simulink model "OPSID_Jawwad"  (R2023a)
settings: Solver=VariableStepAuto  StartTime=0.0  StopTime=10.0  RelTol=1e-3
values from neighbouring files (symbols this model uses):
  Kd = diag([30,30,20,20,20,20])    [parameters.m]
  Kp = diag([280,280,70,70,70,70])    [parameters.m]
libraries: robotcorelib x1
settings Model: Creator=uzair  LastModifiedBy=syedj
settings OptimizationCC: ReuseModelBlockBuffer=off

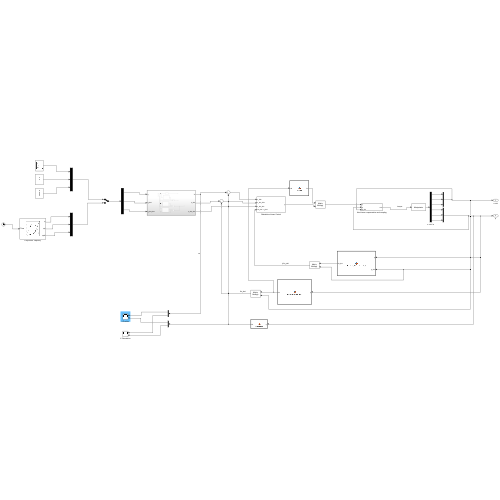
[thumbnail: Simulink's stored preview of the top-level diagram]
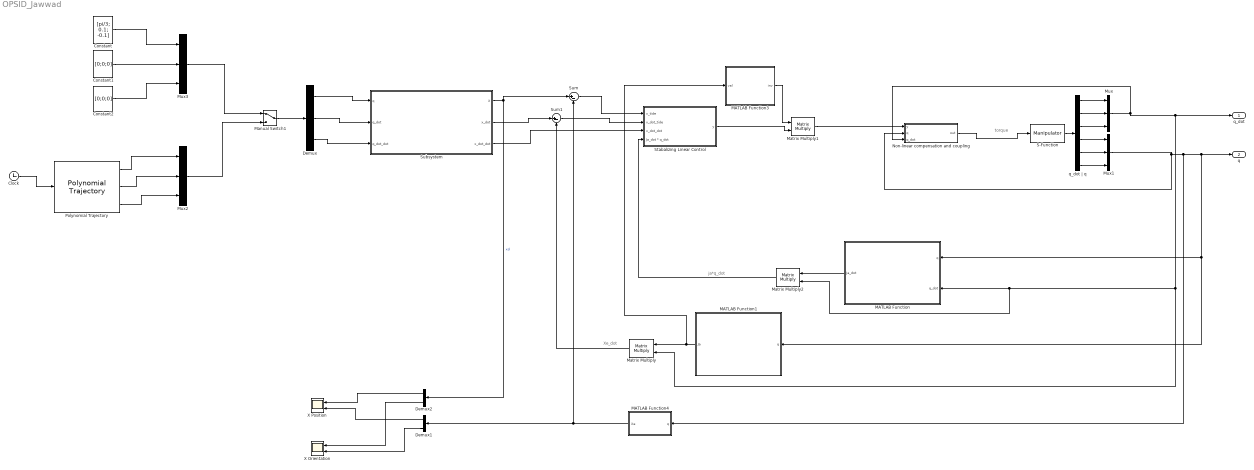
== system OPSID_Jawwad ==
  note: torque
  note: ja*q_dot
  note: Xe_dot
  Clock : Clock
  Constant : Constant  Value=[pi/3; 0.1; -0.1]  VectorParams1D=off
  Constant1 : Constant  Value=[0;0;0]  VectorParams1D=off
  Constant2 : Constant  Value=[0;0;0]  VectorParams1D=off
  Demux : Demux  Outputs=3
  Demux1 : Demux  Outputs=2
  Demux2 : Demux  Outputs=2
  MATLAB Function : MATLAB Function  TreatAsAtomicUnit=on
  MATLAB Function1 : MATLAB Function  TreatAsAtomicUnit=on
  MATLAB Function3 : MATLAB Function  TreatAsAtomicUnit=on
  MATLAB Function4 : MATLAB Function  TreatAsAtomicUnit=on
  Manual Switch1 : ManualSwitch
  Matrix Multiply : Product  Multiplication=Matrix(*)
  Matrix Multiply1 : Product  Multiplication=Matrix(*)
  Matrix Multiply2 : Product  Multiplication=Matrix(*)
  Mux{,1..3} (4 alike) : Mux  Inputs=3
  Non-linear compensation and coupling : Subsystem
  Polynomial Trajectory : robotcorelib/Polynomial Trajectory  WaypointSource=Internal  Waypoints=[pi,2*pi,3*pi; -0.2,0,-0.2; pi/2,pi,pi/2]  TimePoints=[ 0, 4, 9]  TimeInterval=[ 1, 4 ]  Method=Cubic Polynomial  ParameterSource=Internal  VelocityBoundaryCondition=zeros( 3,3 )  AccelerationBoundaryCondition=zeros( 3,3 )  SimulateUsing=Interpreted execution
  S-Function : S-Function  FunctionName=Manipulator  Parameters=params  SFunctionDeploymentMode=off  EnableBusSupport=off
  Stabalizing Linear Control : Subsystem
  Subsystem : Subsystem
  Sum : Sum  Inputs=|+-
  Sum1 : Sum  Inputs=|+-
  X Orientation : Scope  NumInputPorts=2
  X Position : Scope  NumInputPorts=2
  q_dot | q : Demux  Outputs=6
  q_dot : Outport
  q : Outport  Port=2
  wires:
  S-Function/1 -> q_dot | q/1
  q_dot | q/1 -> Mux/1
  q_dot | q/2 -> Mux/2
  q_dot | q/3 -> Mux/3
  q_dot | q/6 -> Mux1/3
  q_dot | q/5 -> Mux1/2
  q_dot | q/4 -> Mux1/1
  Mux/1 -> Matrix Multiply/2, Matrix Multiply2/2, MATLAB Function/2(q_dot), q_dot/1, Non-linear compensation and coupling/3(q_dot)
  Mux1/1 -> Non-linear compensation and coupling/2(q), MATLAB Function4/1(q), MATLAB Function1/1(q), MATLAB Function/1(q), q/1
  Sum/1 -> Stabalizing Linear Control/1(x_tide)
  Sum1/1 -> Stabalizing Linear Control/2(x_dot_tide)
  Clock/1 -> Polynomial Trajectory/1
  Non-linear compensation and coupling/1(out) -> S-Function/1
  Polynomial Trajectory/1 -> Mux2/1
  Polynomial Trajectory/2 -> Mux2/2
  Polynomial Trajectory/3 -> Mux2/3
  Constant/1 -> Mux3/1
  Constant1/1 -> Mux3/2
  Constant2/1 -> Mux3/3
  Mux3/1 -> Manual Switch1/1
  Mux2/1 -> Manual Switch1/2
  Manual Switch1/1 -> Demux/1
  Subsystem/2(x_dot) -> Sum1/1
  Subsystem/3(x_dot_dot) -> Stabalizing Linear Control/3(x_dot_dot)
  Demux/1 -> Subsystem/1(q)
  Demux/2 -> Subsystem/2(q_dot)
  Demux/3 -> Subsystem/3(q_dot_dot)
  MATLAB Function1/1(Ja) -> MATLAB Function3/1(val), Matrix Multiply/1
  Matrix Multiply/1 -> Sum1/2
  Stabalizing Linear Control/1(y) -> Matrix Multiply1/2
  Matrix Multiply1/1 -> Non-linear compensation and coupling/1(y)
  MATLAB Function3/1(inv) -> Matrix Multiply1/1
  MATLAB Function/1(Ja_dot) -> Matrix Multiply2/1
  Matrix Multiply2/1 -> Stabalizing Linear Control/4(Ja_dot * q_dot)
  Demux1/2 -> X Orientation/2
  Demux2/2 -> X Orientation/1
  MATLAB Function4/1(Xe) -> Sum/2, Demux1/1
  Subsystem/1(X) -> Sum/1, Demux2/1  "xd"
  Demux2/1 -> X Position/1
  Demux1/1 -> X Position/2

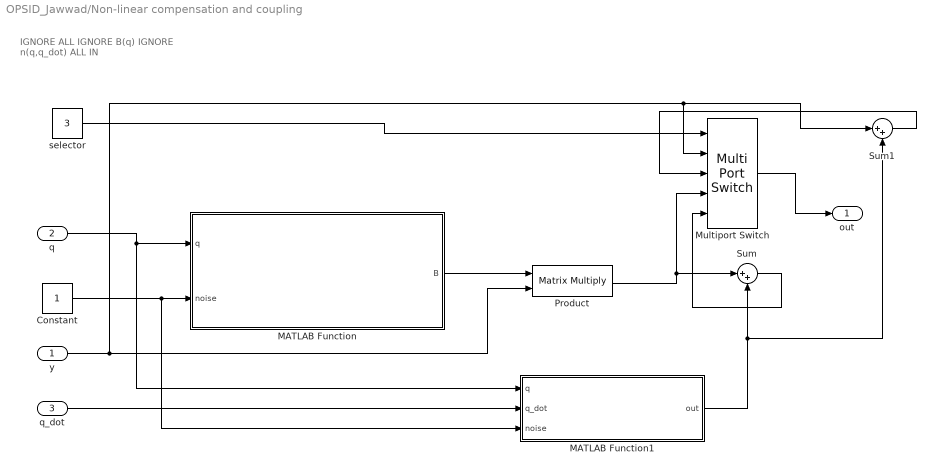
== system OPSID_Jawwad/Non-linear compensation and coupling ==
  note: IGNORE ALL
      | IGNORE B(q)
      | IGNORE n(q,q_dot)
      | ALL IN
  y : Inport
  q : Inport  Port=2
  q_dot : Inport  Port=3
  Constant : Constant
  MATLAB Function : MATLAB Function  TreatAsAtomicUnit=on
  MATLAB Function1 : MATLAB Function  TreatAsAtomicUnit=on
  Multiport Switch : MultiPortSwitch  Inputs=4  SaturateOnIntegerOverflow=off  InputSameDT=off
  Product : Product  Multiplication=Matrix(*)
  Sum : Sum  Inputs=|++
  Sum1 : Sum  Inputs=|++
  selector : Constant  Value=3
  out : Outport
  wires:
  q/1 -> MATLAB Function1/1(q), MATLAB Function/1(q)
  MATLAB Function/1(B) -> Product/1
  y/1 -> Sum1/1, Multiport Switch/2, Product/2
  Product/1 -> Multiport Switch/4, Sum/1
  q_dot/1 -> MATLAB Function1/2(q_dot)
  MATLAB Function1/1(out) -> Sum1/2, Sum/2
  Constant/1 -> MATLAB Function1/3(noise), MATLAB Function/2(noise)
  selector/1 -> Multiport Switch/1
  Multiport Switch/1 -> out/1
  Sum1/1 -> Multiport Switch/3
  Sum/1 -> Multiport Switch/5

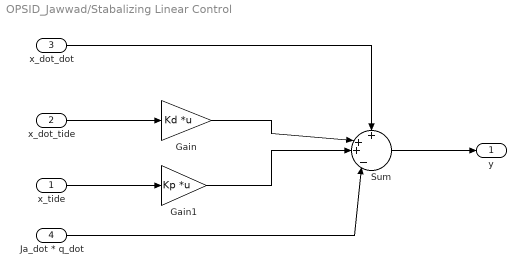
== system OPSID_Jawwad/Stabalizing Linear Control ==
  x_tide : Inport
  x_dot_tide : Inport  Port=2
  x_dot_dot : Inport  Port=3
  Ja_dot * q_dot : Inport  Port=4
  Gain : Gain  Gain=Kd  Multiplication=Matrix(K*u)
  Gain1 : Gain  Gain=Kp  Multiplication=Matrix(K*u)
  Sum : Sum  Inputs=+|++|-|
  y : Outport
  wires:
  x_tide/1 -> Gain1/1
  x_dot_dot/1 -> Sum/1
  Gain1/1 -> Sum/3
  Sum/1 -> y/1
  x_dot_tide/1 -> Gain/1
  Gain/1 -> Sum/2
  Ja_dot * q_dot/1 -> Sum/4

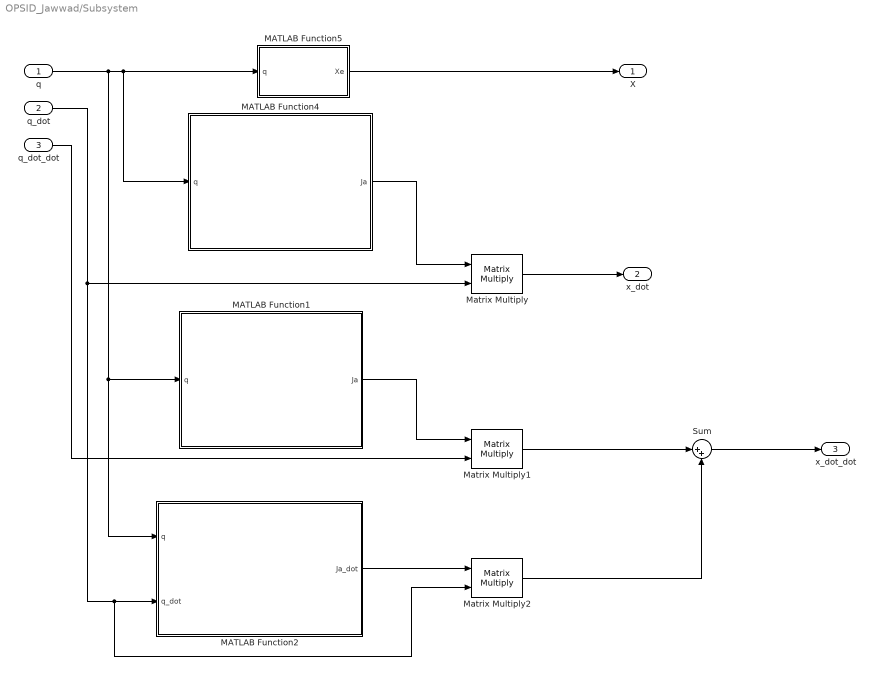
== system OPSID_Jawwad/Subsystem ==
  q : Inport
  q_dot : Inport  Port=2
  q_dot_dot : Inport  Port=3
  MATLAB Function1 : MATLAB Function  TreatAsAtomicUnit=on
  MATLAB Function2 : MATLAB Function  TreatAsAtomicUnit=on
  MATLAB Function4 : MATLAB Function  TreatAsAtomicUnit=on
  MATLAB Function5 : MATLAB Function  TreatAsAtomicUnit=on
  Matrix Multiply : Product  Multiplication=Matrix(*)
  Matrix Multiply1 : Product  Multiplication=Matrix(*)
  Matrix Multiply2 : Product  Multiplication=Matrix(*)
  Sum : Sum  Inputs=|++
  X : Outport
  x_dot : Outport  Port=2
  x_dot_dot : Outport  Port=3
  wires:
  q/1 -> MATLAB Function2/1(q), MATLAB Function1/1(q), MATLAB Function4/1(q), MATLAB Function5/1(q)
  MATLAB Function5/1(Xe) -> X/1
  Matrix Multiply/1 -> x_dot/1
  q_dot/1 -> MATLAB Function2/2(q_dot), Matrix Multiply2/2, Matrix Multiply/2
  MATLAB Function4/1(Ja) -> Matrix Multiply/1
  MATLAB Function1/1(Ja) -> Matrix Multiply1/1
  q_dot_dot/1 -> Matrix Multiply1/2
  Matrix Multiply1/1 -> Sum/1
  Sum/1 -> x_dot_dot/1
  MATLAB Function2/1(Ja_dot) -> Matrix Multiply2/1
  Matrix Multiply2/1 -> Sum/2

== matlab function OPSID_Jawwad/Non-linear compensation and coupling/MATLAB Function1 ==
  data: q input; out output; q_dot input; params parameter; noise input
function out = n(q, q_dot, params, noise)
    
    m1 = params.m(1) * noise;
    m2 = params.m(2) * noise;
    m3 = params.m(3) * noise;

    q1 = q(1);
    q2 = q(2);
    q3 = q(3);

    q1_dot = q_dot(1);
    q2_dot = q_dot(2);
    q3_dot = q_dot(3);

    g = params.g;

    Fv = params.Fv;
 
    r1 = 0.4;
    a1 = 0.02;
    a2 = 0.03;
    a3 = 0.01;
    b1 = 0.1256;
    b2 = 0.03;
    b3 = 0.01;
    c1 = 0.4;
    c2 = 0.46;
    c3 = 0.15;

B = [[(a2^2*m2)/12 + (3*a1^4*m1)/2 + (a3^2*m3)/12 + (3*b1^4*m1)/2 + (b3^2*m3)/12 + c1^2*m1 + c1^2*m2 + c1^2*m3 + (7*c2^2*m2)/12 + (c3^2*m3)/2 + m3*q3^2 + 3*a1^2*b1^2*m1 - c1*c2*m2 + c1*c3*m3 + 2*c1*m3*q3 + c3*m3*q3,       0,  0]
[                                                                                                                                                                                                               0, m2 + m3,  0]
[                                                                                                                                                                                                               0,       0, m3]];
 

C = [[ (m3*q3_dot*(2*c1 + c3 + 2*q3))/2, 0, (m3*q1_dot*(2*c1 + c3 + 2*q3))/2]
[                                0, 0,                                0]
[-(m3*q1_dot*(2*c1 + c3 + 2*q3))/2, 0,                                0]];
 

G = [(c1*g*m1*cos(q1))/2 + g*m2*cos(q1)*(c1 - c2/2) + g*m3*cos(q1)*(c1 + c3/2 + q3)
        0;
        g*m3*sin(q1)];

    out = C*q_dot + diag(Fv)*q_dot + G;
end

== matlab function OPSID_Jawwad/Non-linear compensation and coupling/MATLAB Function ==
  data: q input; B output; params parameter; noise input
function B = inertiaMatrix(q, params, noise)
    q1 = q(1);
    q2 = q(2);
    q3 = q(3);

    m1 = params.m(1) * noise;
    m2 = params.m(2) * noise;
    m3 = params.m(3) * noise;

    a1 = 0.02;
    a2 = 0.03;
    a3 = 0.01;
    b1 = 0.1256;
    b2 = 0.03;
    b3 = 0.01;
    c1 = 0.4;
    c2 = 0.46;
    c3 = 0.15;

B = [[(a2^2*m2)/12 + (3*a1^4*m1)/2 + (a3^2*m3)/12 + (3*b1^4*m1)/2 + (b3^2*m3)/12 + c1^2*m1 + c1^2*m2 + c1^2*m3 + (7*c2^2*m2)/12 + (c3^2*m3)/2 + m3*q3^2 + 3*a1^2*b1^2*m1 - c1*c2*m2 + c1*c3*m3 + 2*c1*m3*q3 + c3*m3*q3,       0,  0]
[                                                                                                                                                                                                               0, m2 + m3,  0]
[                                                                                                                                                                                                               0,       0, m3]];
 
end

== matlab function OPSID_Jawwad/MATLAB Function ==
  data: q input; Ja_dot output; q_dot input
function Ja_dot = AnalyticalJacobian_Dot(q, q_dot)
q1 = q(1);
q2 = q(2);
q3 = q(3);
q1_dot = q_dot(1);
q2_dot = q_dot(2);
q3_dot = q_dot(3);

    r1 = 0.4;
    a1 = 0.02;
    a2 = 0.03;
    a3 = 0.01;
    b1 = 0.1256;
    b2 = 0.03;
    b3 = 0.01;
    c1 = 0.4;
    c2 = 0.46;
    c3 = 0.15;

    H = [[0, -sin(q1), cos(q1),              cos(q1)*(c1 + c3 + q3)]
[1,        0,       0,                           - c2 - q2]
[0,  cos(q1), sin(q1), r1 + sin(q1)*(c3 + q3) + c1*sin(q1)]
[0,        0,       0,                                   1]];


eulers = rotm2eul(H(1:3,1:3), "ZYZ");

    phi1 = eulers(1);
    phi2 = eulers(2);
    phi3 = eulers(3);

Ja_dot_m = [[-cos(q1)*q1_dot*(c1+c2+c3+q3)-(sin(q1)*q3_dot),  0, -sin(q1)*q1_dot]
            [                              0, 0,       0]
            [         (-sin(q1)*q1_dot*(c1 + c3 + q3))+(cos(q1)*q3_dot),  0, cos(q1)*q1_dot]
            [(cos(phi2)*sin(phi1))/sin(phi2),  0,       0]
            [                     -cos(phi1),  0,       0]
            [           -sin(phi1)/sin(phi2),  0,       0]];

Ja_dot = Ja_dot_m;
end

== matlab function OPSID_Jawwad/Subsystem/MATLAB Function1 ==
  data: q input; Ja output
function Ja = AnalyticalJacobian(q)
    q1 = q(1);
    q2 = q(2);
    q3 = q(3);

    r1 = 0.4;
    a1 = 0.02;
    a2 = 0.03;
    a3 = 0.01;
    b1 = 0.1256;
    b2 = 0.03;
    b3 = 0.01;
    c1 = 0.4;
    c2 = 0.46;
    c3 = 0.15;

    H = [[0, -sin(q1), cos(q1),              cos(q1)*(c1 + c3 + q3)]
[1,        0,       0,                           - c2 - q2]
[0,  cos(q1), sin(q1), r1 + sin(q1)*(c3 + q3) + c1*sin(q1)]
[0,        0,       0,                                   1]
];


eulers = rotm2eul(H(1:3,1:3), "ZYZ");


    phi1 = eulers(1);
    phi2 = eulers(2);
    phi3 = eulers(3); %not used

Ja_m = [[        -sin(q1)*(c1 + c3 + q3),  0, cos(q1)]
[                              0, -1,       0]
[         cos(q1)*(c1 + c3 + q3),  0, sin(q1)]
[(cos(phi2)*sin(phi1))/sin(phi2),  0,       0]
[                     -cos(phi1),  0,       0]
[           -sin(phi1)/sin(phi2),  0,       0]
];


    Ja = Ja_m;
end

== matlab function OPSID_Jawwad/Subsystem/MATLAB Function5 ==
  data: q input; Xe output
function Xe = Kinematics(q)
    q1 = q(1);
    q2 = q(2);
    q3 = q(3);
    
    r1 = 0.4;
    a1 = 0.02;
    a2 = 0.03;
    a3 = 0.01;
    b1 = 0.1256;
    b2 = 0.03;
    b3 = 0.01;
    c1 = 0.4;
    c2 = 0.46;
    c3 = 0.15;
    
 H = [[0, -sin(q1), cos(q1),              cos(q1)*(c1 + c3 + q3)]
[1,        0,       0,                           - c2 - q2]
[0,  cos(q1), sin(q1), r1 + sin(q1)*(c3 + q3) + c1*sin(q1)]
[0,        0,       0,                                   1]];

    eulers = rotm2eul(H(1:3,1:3), "ZYZ");

    Xe = [H(1:3,4); eulers'];
end

== matlab function OPSID_Jawwad/Subsystem/MATLAB Function4 ==
  data: q input; Ja output
function Ja = AnalyticalJacobian(q)
    q1 = q(1);
    q2 = q(2);
    q3 = q(3);

    r1 = 0.4;
    a1 = 0.02;
    a2 = 0.03;
    a3 = 0.01;
    b1 = 0.1256;
    b2 = 0.03;
    b3 = 0.01;
    c1 = 0.4;
    c2 = 0.46;
    c3 = 0.15;

    H = [[0, -sin(q1), cos(q1),              cos(q1)*(c1 + c3 + q3)]
[1,        0,       0,                           - c2 - q2]
[0,  cos(q1), sin(q1), r1 + sin(q1)*(c3 + q3) + c1*sin(q1)]
[0,        0,       0,                                   1]
];


eulers = rotm2eul(H(1:3,1:3), "ZYZ");


    phi1 = eulers(1);
    phi2 = eulers(2);
    phi3 = eulers(3); %not used

Ja_m = [[        -sin(q1)*(c1 + c3 + q3),  0, cos(q1)]
[                              0, -1,       0]
[         cos(q1)*(c1 + c3 + q3),  0, sin(q1)]
[(cos(phi2)*sin(phi1))/sin(phi2),  0,       0]
[                     -cos(phi1),  0,       0]
[           -sin(phi1)/sin(phi2),  0,       0]
];


    Ja = Ja_m;
end

== matlab function OPSID_Jawwad/Subsystem/MATLAB Function2 ==
  data: q input; Ja_dot output; q_dot input
function Ja_dot = AnalyticalJacobian_Dot(q, q_dot)
q1 = q(1);
q2 = q(2);
q3 = q(3);

r1 = 0.4;
a1 = 0.02;
a2 = 0.03;
a3 = 0.01;
b1 = 0.1256;
b2 = 0.03;
b3 = 0.01;
c1 = 0.4;
c2 = 0.46;
c3 = 0.15;

q1_dot = q_dot(1);
q2_dot = q_dot(2);
q3_dot = q_dot(3);

H = [[0, -sin(q1), cos(q1),              cos(q1)*(c1 + c3 + q3)]
[1,        0,       0,                           - c2 - q2]
[0,  cos(q1), sin(q1), r1 + sin(q1)*(c3 + q3) + c1*sin(q1)]
[0,        0,       0,                                   1]];



eulers = rotm2eul(H(1:3,1:3), "ZYZ");


phi1 = eulers(1);
phi2 = eulers(2);
phi3 = eulers(3); %not used

Ja_dot_m = [
[        -cos(q1)*q1_dot*(c1 + c3 + q3)-sin(q1)*q3_dot,  0, -sin(q1)*q1_dot]
[                              0, 0,       0]
[         -sin(q1)*q1_dot*(c1 + c3 + q3)+cos(q1)*q3_dot,  0, cos(q1)*q1_dot]
[(cos(phi2)*sin(phi1))/sin(phi2),  0,       0]
[                     -cos(phi1),  0,       0]
[           -sin(phi1)/sin(phi2),  0,       0]
];

Ja_dot = Ja_dot_m;
end

== matlab function OPSID_Jawwad/MATLAB Function4 ==
  data: q input; Xe output
function Xe = Kinematics(q)
    q1 = q(1);
    q2 = q(2);
    q3 = q(3);


    r1 = 0.4;
    a1 = 0.02;
    a2 = 0.03;
    a3 = 0.01;
    b1 = 0.1256;
    b2 = 0.03;
    b3 = 0.01;
    c1 = 0.4;
    c2 = 0.46;
    c3 = 0.15;

 H = [[0, -sin(q1), cos(q1),              cos(q1)*(c1 + c3 + q3)]
[1,        0,       0,                           - c2 - q2]
[0,  cos(q1), sin(q1), r1 + sin(q1)*(c3 + q3) + c1*sin(q1)]
[0,        0,       0,                                   1]];

    eulers = rotm2eul(H(1:3,1:3), "ZYZ");

    Xe = [H(1:3,4); eulers'];
end

== matlab function OPSID_Jawwad/MATLAB Function3 ==
  data: val input; inv output
function inv = inverse(val)
   inv = pinv(val);
end

== matlab function OPSID_Jawwad/MATLAB Function1 ==
  data: q input; Ja output
function Ja = AnalyticalJacobian(q)
    q1 = q(1);
    q2 = q(2);
    q3 = q(3);

    r1 = 0.4;
    a1 = 0.02;
    a2 = 0.03;
    a3 = 0.01;
    b1 = 0.1256;
    b2 = 0.03;
    b3 = 0.01;
    c1 = 0.4;
    c2 = 0.46;
    c3 = 0.15;

    H = [[0, -sin(q1), cos(q1),              cos(q1)*(c1 + c3 + q3)]
[1,        0,       0,                           - c2 - q2]
[0,  cos(q1), sin(q1), r1 + sin(q1)*(c3 + q3) + c1*sin(q1)]
[0,        0,       0,                                   1]];


eulers = rotm2eul(H(1:3,1:3), "ZYZ");


    phi1 = eulers(1);
    phi2 = eulers(2);
    phi3 = eulers(3);
    a1 = 0.02;
    a2 = 0.03;
    a3 = 0.01;
    b1 = 0.1256;
    b2 = 0.03;
    b3 = 0.01;
    c1 = 0.4;
    c2 = 0.46;
    c3 = 0.15;

Ja_m = [
[        -sin(q1)*(c1 + c3 + q3),  0, cos(q1)]
[                              0, -1,       0]
[         cos(q1)*(c1 + c3 + q3),  0, sin(q1)]
[(cos(phi2)*sin(phi1))/sin(phi2),  0,       0]
[                     -cos(phi1),  0,       0]
[           -sin(phi1)/sin(phi2),  0,       0]
];


    Ja = Ja_m;
end
